simulink model "MatlabS"  (R2020a)
settings: Solver=VariableStepAuto  StartTime=0.0  StopTime=inf  RelTol=1e-3
libraries: xpcutilitieslib x2, xpcrtudplib x2, sldrtlib x1
settings Model: Creator=1  LastModifiedBy=1

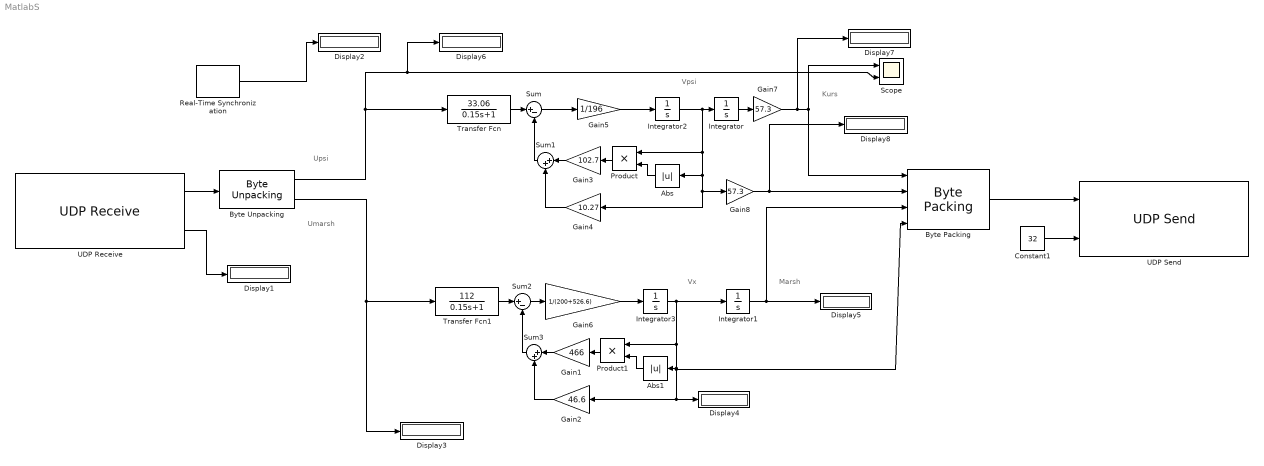
== system MatlabS ==
  note: Vx
  note: Vpsi
  note: Upsi
  note: Umarsh
  note: Marsh
  note: Kurs
  Abs : Abs
  Abs1 : Abs
  "Byte Packing " : xpcutilitieslib/Byte Packing   MaskPackedDataType=uint8  MaskUnpackedDataTypes={'double','double','double','double'}  MaskAlignment=1
  "Byte Unpacking " : xpcutilitieslib/Byte Unpacking   MaskUnpackedDataTypes={'double','double'}  MaskUnpackedDataSizes={[1],[1]}  MaskAlignment=1
      settings: SourceProductBaseCode=XP
  Constant1 : Constant  Value=32
  Display{1..8} (8 alike) : Display
  Gain1 : Gain  Gain=466
  Gain2 : Gain  Gain=46.6
  Gain3 : Gain  Gain=102.7
  Gain4 : Gain  Gain=10.27
  Gain5 : Gain  Gain=1/196
  Gain6 : Gain  Gain=1/(200+526.6)
  Gain7 : Gain  Gain=57.3
  Gain8 : Gain  Gain=57.3
  Integrator{,1..3} (4 alike) : Integrator
  Product : Product
  Product1 : Product
  Real-Time Synchronization : sldrtlib/Real-Time Synchronization  SampleTime=0.01  MaxMissedTicks=10  ShowMissedTicks=on  YieldWhenWaiting=off
  Scope : Scope  NumInputPorts=2
  Sum : Sum  Inputs=|+-
  Sum1 : Sum  Inputs=|++
  Sum2 : Sum  Inputs=|+-
  Sum3 : Sum  Inputs=|++
  Transfer Fcn : TransferFcn  Numerator=[33.06]  Denominator=[0.15 1]
  Transfer Fcn1 : TransferFcn  Numerator=[112]  Denominator=[0.15 1]
  UDP Receive : xpcrtudplib/UDP Receive  ipAddressVal=Use host-target connection  localPort=13042  rcvWidth=16  rcvFmAny=on  fmAddress=0.0.0.0  rcvMulticast=off  multicastAddress={}  maxUDPQueue=8  sampleTime=0.01
  UDP Send : xpcrtudplib/UDP Send  ipAddressVal=Use host-target connection  localPort=13043  toAddress=127.0.0.1  toPort=13044  sampleTime=0.01
      settings: SourceProductBaseCode=XP
  wires:
  UDP Receive/1 -> "Byte Unpacking "/1
  "Byte Packing "/1 -> UDP Send/1
  Constant1/1 -> UDP Send/2
  Transfer Fcn/1 -> Sum/1
  Integrator/1 -> Gain7/1
  Integrator3/1 -> "Byte Packing "/4, Gain2/1, Display4/1, Abs1/1, Product1/1, Integrator1/1
  Integrator1/1 -> Display5/1, "Byte Packing "/3
  Integrator2/1 -> Gain8/1, Gain4/1, Abs/1, Product/1, Integrator/1
  Abs/1 -> Product/2
  Sum1/1 -> Sum/2
  Gain3/1 -> Sum1/1
  Product/1 -> Gain3/1
  Gain4/1 -> Sum1/2
  Sum/1 -> Gain5/1
  Gain5/1 -> Integrator2/1
  Product1/1 -> Gain1/1
  Transfer Fcn1/1 -> Sum2/1
  Sum3/1 -> Sum2/2
  Sum2/1 -> Gain6/1
  Gain1/1 -> Sum3/1
  Abs1/1 -> Product1/2
  Gain6/1 -> Integrator3/1
  Gain2/1 -> Sum3/2
  "Byte Unpacking "/2 -> Transfer Fcn1/1, Display3/1
  Gain7/1 -> Display7/1, "Byte Packing "/1, Scope/1
  Gain8/1 -> Display8/1, "Byte Packing "/2
  "Byte Unpacking "/1 -> Transfer Fcn/1, Display6/1, Scope/2
  UDP Receive/2 -> Display1/1
  Real-Time Synchronization/1 -> Display2/1
